simulink model "r2_deng_tvg"  (R2012b)
(part 3 of 34)

  control_output/1(in_load_en_time) -> pipeline21/1(d)
  bus_create/1(bus_out) -> pipeline29/1(d)
  receptor_id/2(in_pol0_id) -> pipeline30/1(d)
  receptor_id/3(in_pol1_id) -> pipeline31/1(d)
  flag_setup/1(in_adc_count) -> pipeline32/1(d)
  flag_setup/2(in_adc_flag) -> pipeline33/1(d)
  flag_setup/3(in_ndiode_flag) -> pipeline34/1(d)
  flag_setup/4(in_load_flags) -> pipeline35/1(d)
  flag_setup/5(in_reset_flags) -> pipeline36/1(d)
  pipeline36/1(q) -> edge_detect8/1(in)
  pipeline35/1(q) -> edge_detect9/1(in)
  pipeline34/1(q) -> [ndiode_flag]
  pipeline33/1(q) -> [adc_flag]
  pipeline32/1(q) -> [adc_count]
  start_flag_msw/1(in_reg) -> pipeline37/1(d)
  pipeline37/1(q) -> Concat4/1
  start_flag_lsw/1(in_reg) -> pipeline38/1(d)
  pipeline38/1(q) -> Concat4/2
  end_flag_msw/1(in_reg) -> pipeline39/1(d)
  pipeline39/1(q) -> Concat5/1
  end_flag_lsw/1(in_reg) -> pipeline40/1(d)
  pipeline40/1(q) -> Concat5/2
  freq_cwg_corr/1(in_reg) -> pipeline47/1(d)
  pipeline47/1(q) -> cwg_corr/2(scale)
  pipeline53/1(q) -> bus_mult1/1(a)
  pipeline52/1(q) -> bus_mult1/2(b)
  pipeline51/1(q) -> bus_mult/2(b)
  pipeline50/1(q) -> bus_mult/1(a)
  pipeline54/1(q) -> [spead_data0]
  pipeline55/1(q) -> [spead_valid0]
  pipeline56/1(q) -> [spead_eof0]
  pipeline57/1(q) -> [spead_data1]
  pipeline58/1(q) -> [spead_valid1]
  pipeline59/1(q) -> [spead_eof1]
  pipeline60/1(q) -> [spead_data2]
  pipeline61/1(q) -> [spead_valid2]
  pipeline62/1(q) -> [spead_eof2]
  pipeline63/1(q) -> [spead_data3]
  pipeline64/1(q) -> [spead_valid3]
  pipeline65/1(q) -> [spead_eof3]
  [gbe_rst] -> pipeline66/1(d)
  pipeline66/1(q) -> gbe0/1(rst)
  [clr_status] -> pipeline67/1(d)
  pipeline67/1(q) -> gbe0/9(debug_rst)
  pipeline68/1(q) -> gbe1/1(rst)
  pipeline69/1(q) -> gbe1/9(debug_rst)
  pipeline70/1(q) -> gbe2/1(rst)
  pipeline71/1(q) -> gbe2/9(debug_rst)
  [gbe_rst] -> pipeline72/1(d)
  pipeline72/1(q) -> gbe3/1(rst)
  [clr_status] -> pipeline73/1(d)
  pipeline73/1(q) -> gbe3/9(debug_rst)
  pipeline86/1(q) -> gbe0/3(tx_valid)
  pipeline84/1(q) -> gbe0/6(tx_end_of_frame)
  pipeline85/1(q) -> gbe1/3(tx_valid)
  pipeline81/1(q) -> gbe1/6(tx_end_of_frame)
  pipeline82/1(q) -> gbe2/3(tx_valid)
  pipeline87/1(q) -> gbe2/6(tx_end_of_frame)
  pipeline74/1(q) -> gbe3/2(tx_data)
  pipeline75/1(q) -> gbe3/3(tx_valid)
  pipeline76/1(q) -> gbe3/6(tx_end_of_frame)
  pipeline78/1(q) -> bus_addsub/1(a)
  pipeline79/1(q) -> bus_addsub/2(b)
  pipeline88/1(q) -> bus_addsub1/1(a)
  wng_corr/1(bus_out) -> pipeline79/1(d), pipeline88/1(d)
  pipeline89/1(q) -> bus_addsub1/2(b)
  pipeline90/1(q) -> bus_addsub2/1(a)
  pipeline91/1(q) -> bus_addsub2/2(b)
  pipeline92/1(q) -> bus_addsub3/1(a)
  pipeline93/1(q) -> bus_addsub3/2(b)
  pipeline94/1(q) -> [data_80_0]
  pipeline95/1(q) -> [data_80_1]
  pipeline96/1(q) -> pack_80_64_00/1(data80)
  pipeline97/1(q) -> pack_80_64_00/2(valid80)
  pipeline98/1(q) -> pack_80_64_00/3(word_start)
  pipeline99/1(q) -> pack_80_64_00/4(pkt_start)
  pipeline100/1(q) -> pack_80_64_01/1(data80)
  pipeline101/1(q) -> pack_80_64_01/2(valid80)
  pipeline102/1(q) -> pack_80_64_01/3(word_start)
  pipeline103/1(q) -> pack_80_64_01/4(pkt_start)
  pipeline105/1(q) -> pack_80_64_1/2(valid80)
  pipeline104/1(q) -> pack_80_64_1/1(data80)
  pipeline106/1(q) -> pack_80_64_1/3(word_start)
  pipeline107/1(q) -> pack_80_64_1/4(pkt_start)
  pipeline108/1(q) -> pack_80_64_2/1(data80)
  pipeline109/1(q) -> pack_80_64_2/2(valid80)
  pipeline110/1(q) -> pack_80_64_2/3(word_start)
  pipeline111/1(q) -> pack_80_64_2/4(pkt_start)
  pipeline112/1(q) -> spead_pack0/1(data64_ready)
  pipeline113/1(q) -> spead_pack0/2(data64_valid)
  pipeline114/1(q) -> spead_pack0/3(data64)
  pipeline115/1(q) -> spead_pack1/1(data64_ready)
  pipeline116/1(q) -> spead_pack1/2(data64_valid)
  pipeline117/1(q) -> spead_pack1/3(data64)
  pipeline118/1(q) -> spead_pack2/1(data64_ready)
  pipeline119/1(q) -> spead_pack2/2(data64_valid)
  pipeline120/1(q) -> spead_pack2/3(data64)
  pipeline121/1(q) -> spead_pack3/1(data64_ready)
  pipeline122/1(q) -> spead_pack3/2(data64_valid)
  pipeline123/1(q) -> spead_pack3/3(data64)
  pipeline125/1(q) -> [gbe_port2]
  pipeline124/1(q) -> [gbe_port3]
  pipeline15/1(q) -> pipeline14/1(d), pipeline9/1(d)
  Delay2/1 -> bus_addsub4/2(b)
  Delay12/1 -> [status3]
  Delay11/1 -> [status2]
  Delay10/1 -> [status1]
  Delay13/1 -> Logical8/1, Logical6/1
  Delay14/1 -> Logical7/2
  Delay15/1 -> Delay18/1
  Delay16/1 -> Delay19/1
  Delay17/1 -> Logical5/1
  Delay18/1 -> Delay20/1
  Delay19/1 -> Delay21/1
  Delay20/1 -> sample_masking/3(first_samples)
  Delay21/1 -> sample_masking/4(last_samples)
  Delay22/1 -> Logical3/2
  Delay23/1 -> Logical1/1
  Delay24/1 -> Delay25/1
  Delay25/1 -> Delay26/1
  Delay26/1 -> Delay27/1
  Delay27/1 -> sample_masking/1(timei)
  sample_masking/4(flag_valid) -> Delay28/1
  Delay28/1 -> [flag_en]
  Logical1/1 -> sample_masking/7(flag_en)  "flag_en"
  sample_masking/1(timeo) -> Delay29/1
  Delay29/1 -> [masked_time]
  [local_time] -> Delay30/1
  [en_armed] -> Delay31/1
  [local_time] -> Delay32/1, Delay34/1, Delay38/1, Delay40/1
  [start_time] -> Delay33/1
  [end_time] -> Delay35/1, Delay36/1
  Delay30/1 -> Delay24/1
  Delay31/1 -> Delay13/1
  Delay32/1 -> Relational3/1
  Delay33/1 -> Relational3/2
  Delay34/1 -> Relational4/1
  Delay35/1 -> Relational4/2
  Delay36/1 -> Relational5/1
  Delay37/1 -> Relational5/2
  Delay38/1 -> Relational6/1
  Delay39/1 -> Relational6/2
  Delay40/1 -> Relational7/1
  Delay41/1 -> Relational7/2
  Delay44/1 -> Logical4/1, Logical2/1
  Delay45/1 -> Relational/1
  Delay46/1 -> Relational/2
  Delay47/1 -> Relational1/1
  Delay48/1 -> Relational1/2
  Delay51/1 -> Relational2/1
  bus_convert/1(dout) -> pipeline94/1(d)
  bus_convert1/1(dout) -> pipeline95/1(d)
